simulink model "EV_Predictive_Cooling_Plant_Preview"  (R2024b)
settings: Solver=VariableStepAuto  StartTime=0.0  StopTime=1369  RelTol=1e-3
libraries: fl_lib x12, nesl_utility x4, SimscapeFluids_lib x1
settings Model: Creator=HP  LastModifiedBy=HP

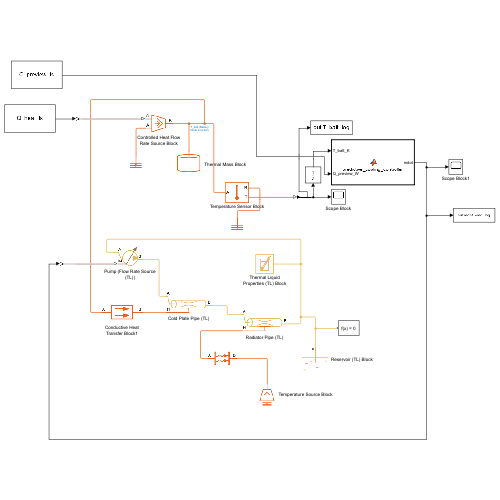
[thumbnail: Simulink's stored preview of the top-level diagram]
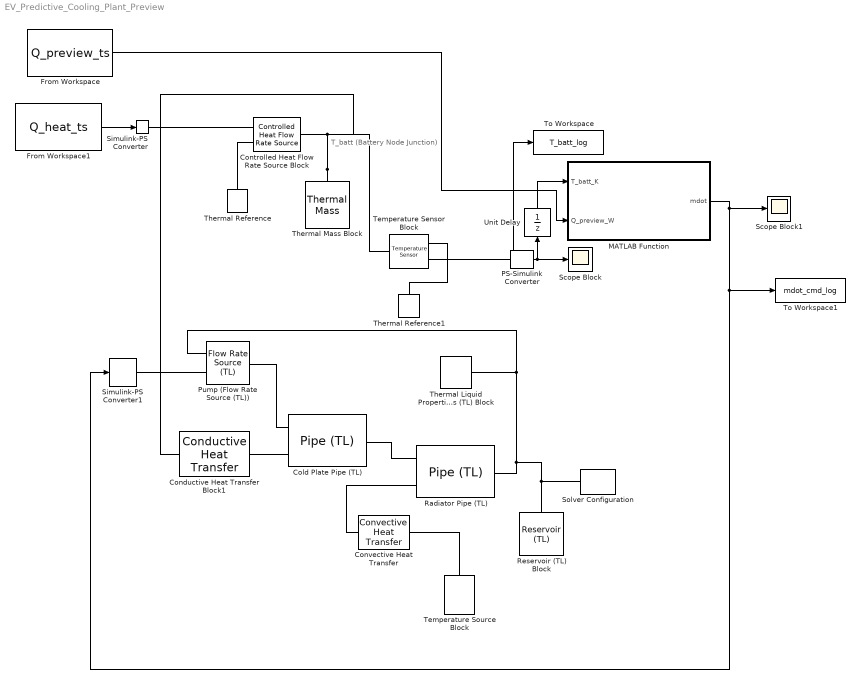
== system EV_Predictive_Cooling_Plant_Preview ==
  note: T_batt (Battery Node Junction)
  Cold Plate Pipe (TL) : fl_lib/Thermal Liquid/Elements/Pipe (TL)  length=2 m  area=1.767e-4 m^2  Dh=0.015 m  length_add=1 m  roughness=15e-6 m  Re_lam=2000  Re_tur=4000  shape_factor=64  Nu_lam=3.66  dynamic_compressibility=true  inertia=false  p0=0.101325 MPa  T0=293.15 K  mdot0=0 kg/s
  Conductive Heat Transfer Block1 : fl_lib/Thermal/Thermal Elements/Conductive Heat Transfer  thermal_type=foundation.enum.ConstantVariableTabulated.Constant  wall_geometry=foundation.enum.ConductionWallGeometry.Planar  area=0.5 m^2  thickness=0.005 m  d_in=0.05 m  d_out=0.1 m  L=1 m  th_cond_min=10 W/(K*m)  th_cond=200 W/(K*m)  th_cond_TLU=[413, 401, 392, 383, 371, 357, 342] W/(K*m)  temp_TLU=[200, 273, 400, 600, 800, 1000, 1200] K  T_specify=off  T_priority=None  T=0 K  T_nominal_specify=off  T_nominal_value=1  T_nominal_unit=K  Q_specify=off  Q_priority=None  Q=0 W  Q_nominal_specify=off  Q_nominal_value=1  Q_nominal_unit=W
  Controlled Heat Flow Rate Source Block : fl_lib/Thermal/Thermal Sources/Controlled Heat Flow Rate Source
  Convective Heat Transfer : fl_lib/Thermal/Thermal Elements/Convective Heat Transfer  thermal_type=foundation.enum.constant_variable.constant  area=1e-4 m^2  heat_tr_coeff=20 W/(K*m^2)  min_heat_tr_coeff=1e-3 W/(K*m^2)  T_specify=off  T_priority=None  T=0 K  T_nominal_specify=off  T_nominal_value=1  T_nominal_unit=K  Q_specify=off  Q_priority=None  Q=0 W  Q_nominal_specify=off  Q_nominal_value=1  Q_nominal_unit=W
  From Workspace : FromWorkspace  VariableName=Q_preview_ts  SampleTime=1
  From Workspace1 : FromWorkspace  VariableName=Q_heat_ts
  MATLAB Function : MATLAB Function  TreatAsAtomicUnit=on  SystemSampleTime=1
  PS-Simulink Converter : nesl_utility/PS-Simulink Converter  PhysicalDomain=network_engine_domain  SubClassName=ps_output  LeftPortType=input  RightPortType=output  PseudoPeriodic=off  Frequencies=[]  VectorFormat=inherit  Unit=K  AffineConversion=off
  Pump (Flow Rate Source (TL)) : fl_lib/Thermal Liquid/Sources/Flow Rate Source (TL)  source_type=foundation.enum.constant_controlled.controlled  flow_type=foundation.enum.mass_volumetric_flow.mass  mass_flow=0 kg/s  volumetric_flow=0 m^3/s  power_spec=foundation.enum.power_spec.isentropic  area=1.767e-4 m^2
  Radiator Pipe (TL) : fl_lib/Thermal Liquid/Elements/Pipe (TL)  length=3 m  area=1.767e-4 m^2  Dh=0.015 m  length_add=1 m  roughness=15e-6 m  Re_lam=2000  Re_tur=4000  shape_factor=64  Nu_lam=3.66  dynamic_compressibility=true  inertia=false  p0=0.101325 MPa  T0=293.15 K  mdot0=0 kg/s
  Reservoir (TL) Block : fl_lib/Thermal Liquid/Elements/Reservoir (TL)  pressure_spec=foundation.enum.pressure_spec.atmospheric  reservoir_pressure=0.101325 MPa  reservoir_temperature=293.15 K  area=0.01 m^2
  Scope Block : Scope
  Scope Block1 : Scope
  Simulink-PS Converter : nesl_utility/Simulink-PS Converter  PhysicalDomain=network_engine_domain  SubClassName=ps_input  LeftPortType=input  RightPortType=output  PseudoPeriodic=off  Frequencies=[]  NoiseDistribution=none  NoiseParameters=[]  Unit=1  AffineConversion=off  FilteringAndDerivatives=provide  SimscapeFilterOrder=1  InputFilterTimeConstant=0.001  UdotUserProvided=0
  Simulink-PS Converter1 : nesl_utility/Simulink-PS Converter  PhysicalDomain=network_engine_domain  SubClassName=ps_input  LeftPortType=input  RightPortType=output  PseudoPeriodic=off  Frequencies=[]  NoiseDistribution=none  NoiseParameters=[]  Unit=kg/s  AffineConversion=off  FilteringAndDerivatives=provide  SimscapeFilterOrder=1  InputFilterTimeConstant=0.001  UdotUserProvided=0
  Solver Configuration : nesl_utility/Solver Configuration  PhysicalDomain=network_engine_domain  SubClassName=solver  LeftPortType=input  RightPortType=generic  Tones=[]  Harmonics=[]  SimulateNoise=off  Profile=off  UseLocalSampling=off  EnableSwitchedLinearOptims=on  FrequencyDomain=off  UseCCode=off  RelTol=0.001  AbsTol=0.001  MinStep=1e-09  ToWorkspace=off  RevertToSquareIcSolve=off  NumHomotopyIterations=100  PhasorMode=off  PhasorModeNumHarmonics=1  ConsistencySolver=NEWTON_XTOL_AFTER_FTOL  IndexReductionMethod=DerivativeReplacement  DoDC=off  ResidualTolerance=1e-09  ConsistencyTolSource=GLOBAL  ConsistencyAbsTol=0.001  ConsistencyRelTol=0.001  ConsistencyTolFactor=0.001  UseLocalSolver=off  LocalSolverChoice=NE_BACKWARD_EULER_ADVANCER  ResolveIndetEquations=on  FunctionEvalNumThread=1  LocalSolverSampleTime=0.001  DoFixedCost=off  MaxNonlinIter=3  MaxModeIter=2  ComputeImpulses=off  ImpulseIterations=2  LinearAlgebra=auto  LinearAlgebraNumThread=0  EquationFormulation=NE_TIME_EF  DelaysMemoryBudget=1024  AutomaticFiltering=on  FilteringTimeConstant=0.001  PartitionStorageMethod=AS_NEEDED  PartitionMemoryBudget=1024  PartitionMethod=ROBUST  MultibodyUseLocalSolver=off  MultibodyLocalSolverChoice=ODE1  MultibodyLocalSolverSampleTime=0.001
  Temperature Sensor Block : fl_lib/Thermal/Thermal Sensors/Temperature Sensor  temperature_measure=foundation.enum.MeasurementReference.difference
  Temperature Source Block : fl_lib/Thermal/Thermal Sources/Temperature Source  temperature=298.15 K
  Thermal Liquid Properties (TL) Block : SimscapeFluids_lib/Thermal Liquid/Utilities/Thermal Liquid Properties (TL)  fluid_list=fluids.thermal_liquid.utilities.enum.thermal_liquid_fluid_list.water  concentration_param_EG=fluids.thermal_liquid.utilities.enum.thermal_liquid_concentration.volume_fraction  concentration_param_PG=fluids.thermal_liquid.utilities.enum.thermal_liquid_concentration.volume_fraction  c_mass_SW=3.5e-3  c_mass_EG=0.1  c_mass_PG=0.1  c_mass_GL=0.1  c_vol_EG=0.1  c_vol_PG=0.1  beta_const_EG=2.1791 GPa  beta_const_PG=2.1791 GPa  beta_const_GL=2.1791 GPa  p_min_EG=0.01 MPa  p_min_PG=0.01 MPa  p_min_GL=0.01 MPa  p_max_EG=50 MPa  p_max_PG=50 MPa  p_max_GL=50 MPa  p_atm=0.101325 MPa  properties_range_check=simscape.enum.assert.action.error
  Thermal Mass Block : fl_lib/Thermal/Thermal Elements/Thermal Mass  mass_type=foundation.enum.constant_variable.constant  mass=180 kg  sp_heat=900 J/(K*kg)  mass_min=1e-6 kg  num_ports=foundation.enum.numPorts2.one  m_specify=off  m_priority=High  m=1 kg  m_nominal_specify=off  m_nominal_value=1  m_nominal_unit=kg  T_specify=off  T_priority=High  T=300 K  T_nominal_specify=off  T_nominal_value=1  T_nominal_unit=K  Q_specify=off  Q_priority=None  Q=0 W  Q_nominal_specify=off  Q_nominal_value=1  Q_nominal_unit=W
  Thermal Reference : fl_lib/Thermal/Thermal Elements/Thermal Reference
  Thermal Reference1 : fl_lib/Thermal/Thermal Elements/Thermal Reference
  To Workspace : ToWorkspace  VariableName=T_batt_log  SaveFormat=Timeseries  SampleTime=-1
  To Workspace1 : ToWorkspace  VariableName=mdot_cmd_log  SaveFormat=Timeseries  SampleTime=-1
  Unit Delay : UnitDelay  HasFrameUpgradeWarning=on
  wires:
  PS-Simulink Converter/1 -> To Workspace/1, Scope Block/1, Unit Delay/1
  MATLAB Function/1(mdot) -> To Workspace1/1, Simulink-PS Converter1/1, Scope Block1/1
  Unit Delay/1 -> MATLAB Function/1(T_batt_K)
  From Workspace/1 -> MATLAB Function/2(Q_preview_W)
  From Workspace1/1 -> Simulink-PS Converter/1
  connections:
  Reservoir (TL) Block/LConn1 -- Radiator Pipe (TL)/RConn1 -- Thermal Liquid Properties (TL) Block/RConn1 -- Pump (Flow Rate Source (TL))/LConn1 -- Solver Configuration/RConn1
  Thermal Mass Block/LConn1 -- Controlled Heat Flow Rate Source Block/LConn1 -- Temperature Sensor Block/LConn1 -- Conductive Heat Transfer Block1/LConn1
  Conductive Heat Transfer Block1/RConn1 -- Cold Plate Pipe (TL)/LConn2
  Simulink-PS Converter1/RConn1 -- Pump (Flow Rate Source (TL))/LConn2
  Radiator Pipe (TL)/LConn2 -- Convective Heat Transfer/LConn1
  Pump (Flow Rate Source (TL))/RConn1 -- Cold Plate Pipe (TL)/LConn1
  Controlled Heat Flow Rate Source Block/RConn2 -- Thermal Reference/LConn1
  Temperature Sensor Block/RConn1 -- Thermal Reference1/LConn1
  Cold Plate Pipe (TL)/RConn1 -- Radiator Pipe (TL)/LConn1
  Temperature Sensor Block/RConn2 -- PS-Simulink Converter/LConn1
  Convective Heat Transfer/RConn1 -- Temperature Source Block/LConn1
  Simulink-PS Converter/RConn1 -- Controlled Heat Flow Rate Source Block/RConn1

== matlab function EV_Predictive_Cooling_Plant_Preview/MATLAB Function ==
  data: T_batt_K input; mdot output; Q_preview_W input
function mdot = predictive_cooling_controller(T_batt_K,Q_preview_W)
% Preview-triggered predictive cooling controller
% T_batt_K: measured battery temperature
% Q_preview_W: maximum predicted heat generation in next 60 s
% mdot: coolant mass flow command in kg/s

persistent coolingOn

if isempty(coolingOn)
    coolingOn = false;
end

% Controller thresholds
T_on_K  = 32 + 273.15;
T_off_K = 30 + 273.15;

% Preview horizon and battery thermal capacitance
preview_horizon_s = 60;
C_th = 45000;       % J/K

% Flow limits
mdot_low  = 0.005;  % kg/s
mdot_high = 0.050;  % kg/s

% Conservative temperature prediction
Q_predicted_W = max(Q_preview_W,0);
T_predicted_K = T_batt_K + ...
    Q_predicted_W*preview_horizon_s/C_th;

% Turn cooling on using present or predicted temperature
if ~coolingOn && ...
        (T_batt_K >= T_on_K || T_predicted_K >= T_on_K)
    coolingOn = true;
elseif coolingOn && T_batt_K <= T_off_K
    coolingOn = false;
end

if coolingOn
    mdot = mdot_high;
else
    mdot = mdot_low;
end
